simulink model "ASK_1"  (R2017b)
settings: Solver=VariableStepAuto  StartTime=0.0  StopTime=10.0  MaxStep=0.01  MinStep=0.001  RelTol=1e-3
libraries: dsparch4 x1
settings Model: Creator=ayadd  LastModifiedBy=ayadd
settings SolverCC: ShapePreserveControl=EnableAll  ZeroCrossAlgorithm=Adaptive

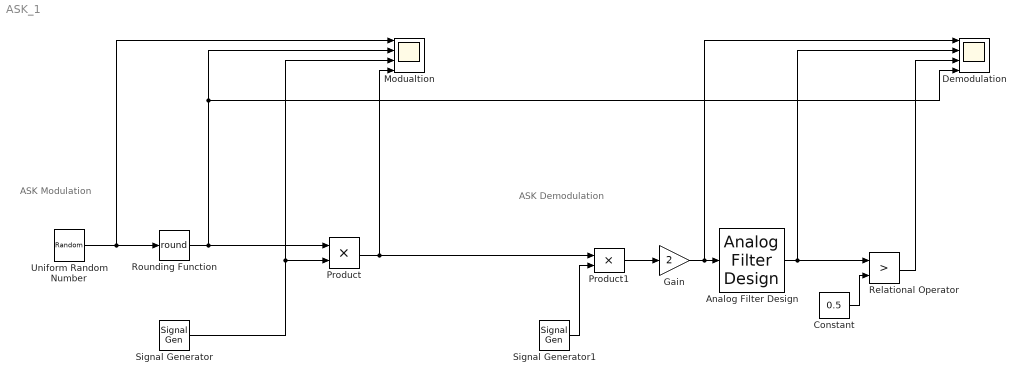
== system ASK_1 ==
  note: ASK Demodulation
  note: ASK Modulation
  Analog Filter Design : dsparch4/Analog Filter Design  method=Butterworth  filttype=Lowpass  N=8  Wlo=30  Whi=80  Rp=2  Rs=40
  Constant : Constant  Value=0.5
  Demodulation : Scope  NumInputPorts=4
  Gain : Gain  Gain=2
  Modualtion : Scope  NumInputPorts=4
  Product : Product
  Product1 : Product  SaturateOnIntegerOverflow=on  InputSameDT=on  OutDataTypeStr=Inherit: Same as first input
  Relational Operator : RelationalOperator  Operator=>  RndMeth=Nearest  InputSameDT=on
  Rounding Function : Rounding  Operator=round
  Signal Generator : SignalGenerator  Frequency=4
  Signal Generator1 : SignalGenerator  Frequency=4
  Uniform Random Number : UniformRandomNumber  Minimum=0  SampleTime=1
  wires:
  Uniform Random Number/1 -> Modualtion/1, Rounding Function/1
  Signal Generator/1 -> Modualtion/3, Product/2
  Signal Generator1/1 -> Product1/2
  Product/1 -> Modualtion/4, Product1/1
  Product1/1 -> Gain/1
  Analog Filter Design/1 -> Demodulation/2, Relational Operator/1
  Constant/1 -> Relational Operator/2
  Gain/1 -> Demodulation/1, Analog Filter Design/1
  Relational Operator/1 -> Demodulation/3
  Rounding Function/1 -> Modualtion/2, Demodulation/4, Product/1
